simulink model "FuzzyHYPFWMLI"  (R2025a)
settings: Solver=ode23t  StartTime=0.0  StopTime=1  FixedStep=1.0000000100000003E-5  MaxStep=1e-3  RelTol=1e-2  EnableMultiTasking=on
undefined symbols (not defined in the file): c1, c2, c3, c4, c5, c6, DiscIntNeverNeededParam, FC1, FC2, idq1, idq2, PV10k1, PV10k2, PV10k3, R, WM1
libraries: powerlib x93, powerlib_meascontrol x9, fuzblock x8, powerlib_extras x6, re_lib x3, electricdrivelib x2, slpidlib x1
(part 3 of 3)

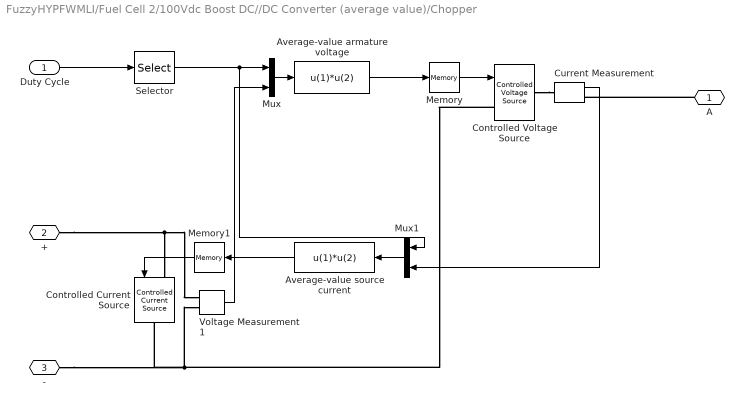
== system FuzzyHYPFWMLI/Fuel Cell 2/100Vdc Boost DC//DC Converter (average value)/Chopper ==
  Duty Cycle : Inport
  Average-value armature voltage : Fcn  Expr=u(1)*u(2)
  Average-value source current : Fcn  Expr=u(1)*u(2)
  Controlled Current Source : powerlib/Electrical Sources/Controlled Current Source  Initialize=on  Source_Type=AC  Amplitude=0  Phase=0  Frequency=0  Measurements=None
  Controlled Voltage Source : powerlib/Electrical Sources/Controlled Voltage Source  Initialize=on  Source_Type=AC  Amplitude=0  Phase=0  Frequency=0  Measurements=None
  Current Measurement : powerlib/Measurements/Current Measurement  Tag=PoWeRsYsTeMmEaSuReMeNt  PhasorSimulation=off  OutputType=Magnitude  PSBequivalent=0
  Memory : Memory
  Memory1 : Memory
  Mux : Mux  Inputs=2
  Mux1 : Mux  Inputs=2
  Selector : Selector  InputPortWidth=2  IndexOptions=Index vector (dialog)  Indices=[1]  OutputSizes=1
  Voltage Measurement1 : powerlib/Measurements/Voltage Measurement  Tag=PoWeRsYsTeMmEaSuReMeNt  PhasorSimulation=off  OutputType=Magnitude  PSBequivalent=0
  A : PMIOPort  Side=Right
  + : PMIOPort  Port=2  Side=Left
  - : PMIOPort  Port=3  Side=Left
  wires:
  Selector/1 -> Mux1/1, Mux/1
  Memory1/1 -> Controlled Current Source/1
  Average-value source current/1 -> Memory1/1
  Current Measurement/1 -> Mux1/2
  Mux1/1 -> Average-value source current/1
  Duty Cycle/1 -> Selector/1
  Voltage Measurement1/1 -> Mux/2
  Mux/1 -> Average-value armature voltage/1
  Average-value armature voltage/1 -> Memory/1
  Memory/1 -> Controlled Voltage Source/1
  connections:
  A/RConn1 -- Current Measurement/RConn1
  Controlled Voltage Source/RConn1 -- Current Measurement/LConn1
  +/RConn1 -- Voltage Measurement1/LConn1 -- Controlled Current Source/LConn1
  Controlled Voltage Source/LConn1 -- -/RConn1 -- Controlled Current Source/RConn1 -- Voltage Measurement1/LConn2

== system FuzzyHYPFWMLI/Fuel Cell 2/100Vdc Boost DC//DC Converter (average value)/Current controller DISCRETE1 ==
  UBus : Inport
  Uref : Inport  Port=2
  Ctrl sat. : Saturate  UpperLimit=0.95  LowerLimit=-0.95
  Discrete-Time Integrator : DiscreteIntegrator  IntegratorMethod=Integration: Trapezoidal  SampleTime=Ts  LimitOutput=on  UpperSaturationLimit=0.95  LowerSaturationLimit=-0.95  ICPrevOutput=DiscIntNeverNeededParam  ICPrevScaledInput=DiscIntNeverNeededParam
  Integral gain : Gain  Gain=Ki  SaturateOnIntegerOverflow=on  OutDataTypeStr=Inherit: Same as input  ParamDataTypeStr=Inherit: Same as input
  Proportional gain : Gain  Gain=Kp  SaturateOnIntegerOverflow=on  OutDataTypeStr=Inherit: Same as input  ParamDataTypeStr=Inherit: Same as input
  Sum1 : Sum  Inputs=+-  InputSameDT=on  SaturateOnIntegerOverflow=on  OutDataTypeStr=Inherit: Same as first input
  Sum2 : Sum  InputSameDT=on  SaturateOnIntegerOverflow=on  OutDataTypeStr=Inherit: Same as first input
  Ec : Outport  InitialOutput=0  VectorParamsAs1DForOutWhenUnconnected=off
  wires:
  Ctrl sat./1 -> Ec/1
  Sum2/1 -> Ctrl sat./1
  Discrete-Time Integrator/1 -> Sum2/2
  Uref/1 -> Sum1/2
  UBus/1 -> Sum1/1
  Sum1/1 -> Proportional gain/1, Integral gain/1
  Integral gain/1 -> Discrete-Time Integrator/1
  Proportional gain/1 -> Sum2/1

== system FuzzyHYPFWMLI/Fuel Cell 2/100Vdc Boost DC//DC Converter (average value)/Duty Cycles ==
  Ec : Inport
  Add : Sum  Inputs=+-
  Bus Creator2 : BusCreator  Inputs=2
  Constant : Constant
  Duty Cycle : Fcn  Expr=0.5*(u[1]+1)
  dc : Outport  VectorParamsAs1DForOutWhenUnconnected=off
  wires:
  Bus Creator2/1 -> dc/1
  Ec/1 -> Duty Cycle/1
  Constant/1 -> Add/1
  Add/1 -> Bus Creator2/2  "IGBT 2"
  Duty Cycle/1 -> Bus Creator2/1, Add/2  "IGBT I"

== system FuzzyHYPFWMLI/Wind  Power /Wind Turbine model1/cp(lambda,beta) ==
  lambda : Inport
  beta : Inport  Port=2
  Fcn : Fcn  Expr=1/(1/(u[1]+0.08*u[2])-0.035/(u[2]^3+1))
  Fcn1 : Fcn  Expr=c1*(c2/u[2]-c3*u[3]-c4)*exp(-c5/u[2])+c6*u[1]
  Mux : Mux  Inputs=2
  Mux1 : Mux  Inputs=3
  cp : Outport  VectorParamsAs1DForOutWhenUnconnected=off
  wires:
  Mux/1 -> Fcn/1
  beta/1 -> Mux/2, Mux1/3
  Mux1/1 -> Fcn1/1
  lambda/1 -> Mux/1, Mux1/1
  Fcn1/1 -> cp/1
  Fcn/1 -> Mux1/2  "lambda_i"
